simulink model "smith_disc"  (Simulink 5.0)
settings: Solver=ode45  StartTime=t_init  StopTime=t_final  RelTol=1e-3
values from neighbouring files (symbols this model uses):
  A = [1 -0.44]    [visc_imc1.m]
  st = 1    [lewin_imc1.m]
  Ts = 3    [lewin_imc1.m]    (also in lewin_imc_general.m; visc_imc1.m = 0.1)
undefined symbols (not defined in the file or in its folder): Bd, C, D, gamma, mzkd, N_var, Rc, Sc, Tc, zkd
settings Model: Creator=kannan  LastModifiedBy=kannan  ExtModeAutoUpdateStatusClock=off

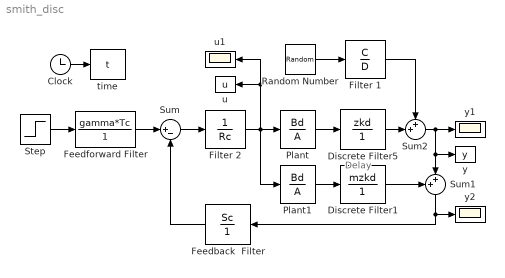
== system smith_disc ==
  note: Delay
  " Filter 2" : DiscreteFilter  Numerator=1  Denominator=Rc  SampleTime=Ts
  Clock : Clock
      settings: Decimation=10
  Discrete Filter1 : DiscreteFilter  Numerator=mzkd  Denominator=1  SampleTime=Ts
  Discrete Filter5 : DiscreteFilter  Numerator=zkd  Denominator=1  SampleTime=Ts
  Feedback  Filter : DiscreteFilter  Orientation=left  Numerator=Sc  Denominator=1  SampleTime=Ts
  Feedforward Filter : DiscreteFilter  Numerator=gamma*Tc  Denominator=1  SampleTime=Ts
  Filter 1 : DiscreteFilter  Numerator=C  Denominator=D  SampleTime=Ts
  Plant : DiscreteFilter  Numerator=Bd  Denominator=A  SampleTime=Ts
  Plant1 : DiscreteFilter  Numerator=Bd  Denominator=A  SampleTime=Ts
  Random Number : RandomNumber  Variance=N_var  SampleTime=Ts
  Step : Step  Time=0  After=st  SampleTime=Ts
  Sum : Sum  Inputs=|+-  SaturateOnIntegerOverflow=on
  Sum1 : Sum  Orientation=down  Inputs=++|  SaturateOnIntegerOverflow=on
  Sum2 : Sum  Inputs=++|  SaturateOnIntegerOverflow=on
  time : ToWorkspace  VariableName=t  SampleTime=Ts  SaveFormat=Array
  u : ToWorkspace  VariableName=u  SampleTime=Ts  SaveFormat=Array
  u1 : Scope
      settings: YMin=-6e+164  YMax=1.02293e+149
  y : ToWorkspace  VariableName=y  SampleTime=Ts  SaveFormat=Array
  y1 : Scope
      settings: YMin=-6e+164  YMax=1.02293e+149
  y2 : Scope
      settings: YMin=-6e+164  YMax=1.02293e+149  SaveName=ScopeData2
  wires:
  Feedforward Filter/1 -> Sum/1
  Feedback  Filter/1 -> Sum/2
  Clock/1 -> time/1
  Plant/1 -> Discrete Filter5/1
  Discrete Filter5/1 -> Sum2/2
  Filter 1/1 -> Sum2/1
  Random Number/1 -> Filter 1/1
  Sum2/1 -> y1/1, y/1, Sum1/2
  Sum/1 -> " Filter 2"/1
  " Filter 2"/1 -> Plant/1, u1/1, u/1, Plant1/1
  Step/1 -> Feedforward Filter/1
  Plant1/1 -> Discrete Filter1/1
  Discrete Filter1/1 -> Sum1/1
  Sum1/1 -> Feedback  Filter/1, y2/1
